simulink model "Syn_Leader_Follower"  (R2022b)
settings: Solver=VariableStepAuto  StartTime=0.0  StopTime=1.5  RelTol=1e-3
settings Model: Creator=JianFongLee  LastModifiedBy=allen
settings DebuggingCC: UnconnectedInputMsg=warning  UnconnectedOutputMsg=warning  UnconnectedLineMsg=warning
settings ModelReferenceCC: EnableRefExpFcnMdlSchedulingChecks=on
settings RTWCC: DLArmComputeVersion=19.05

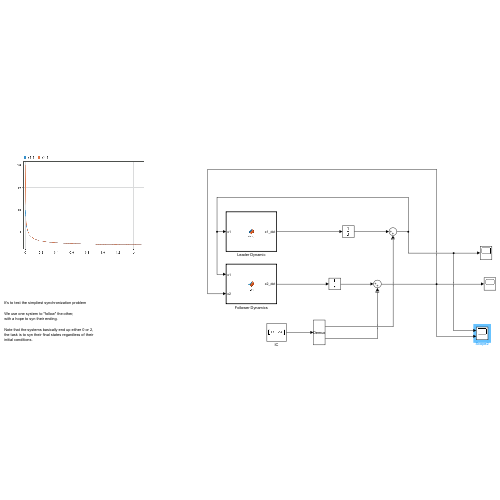
[thumbnail: Simulink's stored preview of the top-level diagram]
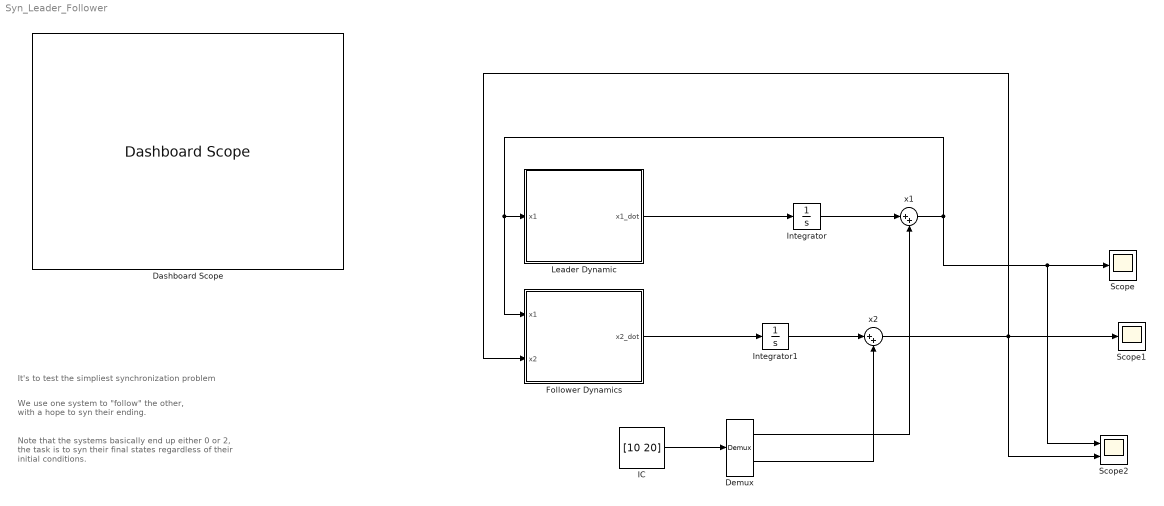
== system Syn_Leader_Follower ==
  note: Note that the systems basically end up either 0 or 2,
      | the task is to syn their final states regardless of their
      | initial conditions.
  note: We use one system to "follow" the other,
      | with a hope to syn their ending.
  note: It's to test the simpliest synchronization problem
  Dashboard Scope : DashboardScope
  Demux : Demux  Outputs=2
      settings: DisplayOption=none
  Follower Dynamics : MATLAB Function  TreatAsAtomicUnit=on
  IC : Constant  Value=[10 20]
  Integrator : Integrator
  Integrator1 : Integrator
  Leader Dynamic : MATLAB Function  TreatAsAtomicUnit=on
  Scope : Scope
  Scope1 : Scope
  Scope2 : Scope  NumInputPorts=2
  x1 : Sum  Inputs=|++
  x2 : Sum  Inputs=|++
  wires:
  Leader Dynamic/1(x1_dot) -> Integrator/1
  Integrator/1 -> x1/1
  x1/1 -> Scope2/1, Scope/1, Follower Dynamics/1(x1), Leader Dynamic/1(x1)
  Follower Dynamics/1(x2_dot) -> Integrator1/1
  IC/1 -> Demux/1
  Demux/1 -> x1/2
  Integrator1/1 -> x2/1
  Demux/2 -> x2/2
  x2/1 -> Scope2/2, Scope1/1, Follower Dynamics/2(x2)

== matlab function Syn_Leader_Follower/Leader Dynamic ==
  data: x1 input; x1_dot output
function x1_dot = fcn(x1)
 
%%% System leader
x1_dot = -x1*(x1-2)*(x1-2);
%%% This system converges to 2 for x > 2,
%%% and converges to 0 for the rest states.

%%% It's a stable system regardless of IC
end

== matlab function Syn_Leader_Follower/Follower Dynamics ==
  data: x1 input; x2_dot output; x2 input
function x2_dot = fcn(x1,x2)
 
%%% System follower, comprising u to syn with x1
u = 4*(x1^2 - x2^2);
x2_dot = -x2*(x2-2)*(x2-2) + u;
%%% With the same dynamics of x1 except u is employed,
%%% so it would follow where x1 ends up in this case.
end
